simulink model "DC_Simscape"  (R2016a)
settings: Solver=ode15s  StartTime=0.0  StopTime=10  RelTol=1e-3
PreLoadFcn:
  | t_sim = 1;
  | T = 25;
libraries: fl_lib x6, nesl_utility x5, simulink x4, elec_lib x1
Description:
  | Schottky Barrier Diode Characteristics
  | 
  | This example shows generation of the current versus voltage curve
  | for a Schottky barrier diode. Define the vector of temperatures for
  | which to plot the characteristics by double clicking on the block
  | labeled 'Define temperatures'. Then double click on the block
  | labeled 'Generate Characteristics'. The datasheet for this device
  | gives Vf = 0.4V when If = 10mA, and Vf = 0.65V when If = 100mA.
  | The ohmic resistance is set to one over the gradient of the
  | datasheet I-V curve at higher voltages. The temperature
  | dependence is then modeled by selecting the default energy gap
  | and saturation current temperature exponent values for a Schottky
  | barrier diode. The plot produced by this test model can be used to
  | validate the implementation against the datasheet I-V plots.
  | 
  | 
  | Copyright 2008-2016 The MathWorks, Inc.
settings Model: ExtModeAutoUpdateStatusClock=off  Creator=MathWorks  LastModifiedBy=sara
settings DataIOCC: LimitDataPoints=on  SaveFormat=Array  SignalLoggingSaveFormat=ModelDataLogs  OutputOption=SpecifiedOutputTimes  OutputTimes=[0:t_sim/4000:t_sim]  Refine=5
settings OptimizationCC: ExpressionDepthLimit=2147483647  InitFltsAndDblsToZero=on
settings DebuggingCC: SaveWithParameterizedLinksMsg=none  UnderspecifiedInitializationDetection=Classic  MergeDetectMultiDrivingBlocksExec=none  SignalResolutionControl=TryResolveAllWithWarning  FcnCallInpInsideContextMsg=UseLocalSettings  StateNameClashWarn=warning
settings HardwareCC: ProdBitPerPointer=32  ProdLargestAtomicFloat=None  ProdIntDivRoundTo=Undefined  ProdEndianess=Unspecified  ProdWordSize=32  ProdHWDeviceType=32-bit Generic
settings ModelReferenceCC: PropagateSignalLabelsOutOfModel=off
settings GRTTargetCC: TargetFcnLib=ansi_tfl_tmw.mat  CombineOutputUpdateFcns=off  GRTInterface=on
settings ConfigComp: CovModelRefEnable=Off  CovSFcnEnable=off

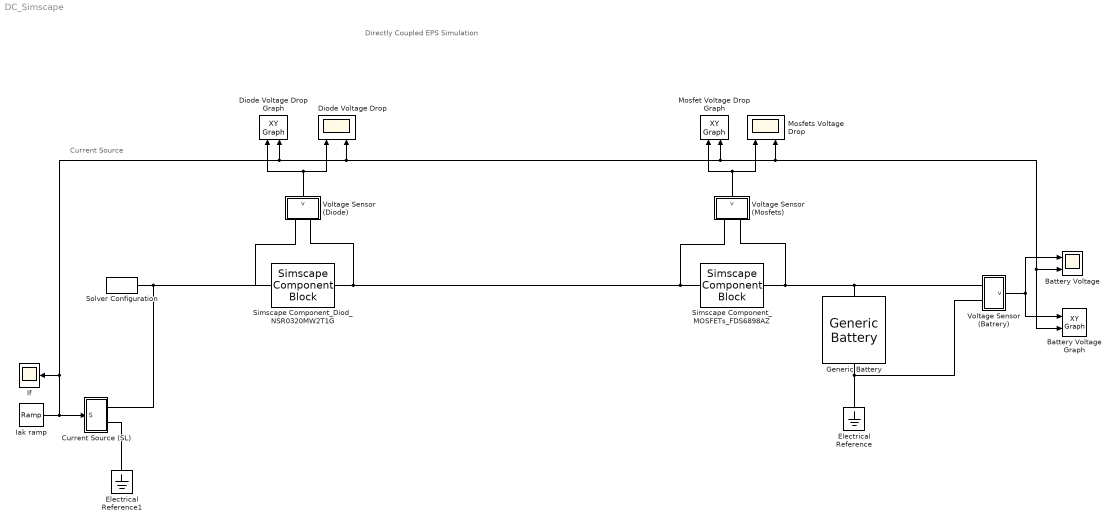
== system DC_Simscape ==
  note: Current Source
  note: Directly Coupled EPS Simulation
  " Mosfet Voltage Drop Graph" : simulink/Sinks/XY Graph  xmin=0  xmax=1  ymin=0  ymax=1  st=-1
  Battery Voltage : Scope  NumInputPorts=2
  Battery Voltage Graph : simulink/Sinks/XY Graph  xmin=0  xmax=10  ymin=0  ymax=3  st=-1
  Current Source (SL) : Subsystem
      settings: CopyFcn=set_param(gcb,'LinkStatus','none')
  Diode Voltage Drop : Scope  NumInputPorts=2
  Diode Voltage Drop Graph : simulink/Sinks/XY Graph  xmin=0  xmax=1  ymin=0  ymax=1  st=-1
  Electrical Reference : fl_lib/Electrical/Electrical Elements/Electrical Reference
  Electrical Reference1 : fl_lib/Electrical/Electrical Elements/Electrical Reference
  Generic Battery : elec_lib/Sources/Generic Battery  Vnom=2 V  R1=2 Ohm  prm_AH=1  AH=50 hr*A  AH0=50 hr*A  V1=11.5 V  AH1=25 hr*A  prm_R2=1  R2=2e+3 Ohm
  Iak ramp : simulink/Sources/Ramp  slope=2  start=0  X0=0.01
  If : Scope
  Mosfets Voltage Drop : Scope  NumInputPorts=2
  Simscape Component_Diod_NSR0320MW2T1G : SimscapeComponentBlock  SourceFile=diode_EPS  ComponentPath=diode_EPS  ComponentVariants=diode_EPS  ComponentVariantNames=diode_EPS  ClassName=diode_EPS  SchemaVersion=1  Vt=1.38e-23 * 298 / 1.60e-19 V  R=0.0084 Ohm  n=1.00404  Is=1.3032e-6 A  i_specify=off  i_priority=None  i=1 A  v_specify=off  v_priority=None  v=0 V
      settings: CopyFcn=simscape.engine.sli.internal.componentblockcallback(gcbh,'COPY')  PreCopyFcn=simscape.engine.sli.internal.componentblockcallback(gcbh,'PRECOPY')  PreDeleteFcn=simscape.engine.sli.internal.componentblockcallback(gcbh,'PREDELETE')
      mask Type: Code produced by Embedded Systems Group - UFSC
      mask Display:
      | disp('Simscape\n\n\n')
      | disp('\n\n\ndiode_EPS');
      | color('red');
      | port_label('RConn', 1,'-');
      | port_label('LConn', 1,'+');
  Simscape Component_MOSFETs_FDS6898AZ : SimscapeComponentBlock  SourceFile=MOSFETs_EPS  ComponentPath=MOSFETs_EPS  ComponentVariants=MOSFETs_EPS  ComponentVariantNames=MOSFETs_EPS  ClassName=MOSFETs_EPS  SchemaVersion=1  Vt=1.38e-23 * 298 / 1.60e-19 V  Rsd=0.27 Ohm  Rs=0.008235 Ohm  n=1.89492  Is=1.26064e-7 A  i_specify=off  i_priority=None  i=1 A  v_specify=off  v_priority=None  v=0 V  Vr_DC_specify=off  Vr_DC_priority=None  Vr_DC=0 V  Vr_CC_specify=off  Vr_CC_priority=None  Vr_CC=0 V
      settings: CopyFcn=simscape.engine.sli.internal.componentblockcallback(gcbh,'COPY')  PreCopyFcn=simscape.engine.sli.internal.componentblockcallback(gcbh,'PRECOPY')  PreDeleteFcn=simscape.engine.sli.internal.componentblockcallback(gcbh,'PREDELETE')
      mask Type: Code produced by Embedded Systems Group - UFSC
      mask Display:
      | disp('Simscape\n\n\n')
      | disp('\n\n\nMOSFETs_EPS');
      | color('red');
      | port_label('RConn', 1,'-');
      | port_label('LConn', 1,'+');
  Solver Configuration : nesl_utility/Solver Configuration  PhysicalDomain=network_engine_domain  SubClassName=solver  LeftPortType=input  RightPortType=generic  Accelerate=off  Tones=[]  Harmonics=[]  SimulateNoise=off  Profile=off  UseLocalSampling=off  EnableSwitchedLinearOptims=on  FrequencyDomain=off  UseCCode=off  RelTol=0.001  AbsTol=1e-06  MinStep=1e-09  ToWorkspace=off  RevertToSquareIcSolve=off  NumHomotopyIterations=100  PhasorMode=off  PhasorModeNumHarmonics=1  OverrideAbsTol=off  DoDC=on  ResidualTolerance=1e-9  UseLocalSolver=off  LocalSolverChoice=NE_BACKWARD_EULER_ADVANCER  LocalSolverSampleTime=.001  DoFixedCost=off  MaxNonlinIter=3  MaxModeIter=2  LinearAlgebra=Sparse  DelaysMemoryBudget=1024  AutomaticFiltering=on  FilteringTimeConstant=0.001
  Voltage Sensor (Batrery) : Subsystem
      settings: CopyFcn=set_param(gcb,'LinkStatus','none')
  Voltage Sensor (Diode) : Subsystem
      settings: CopyFcn=set_param(gcb,'LinkStatus','none')
  Voltage Sensor (Mosfets) : Subsystem
      settings: CopyFcn=set_param(gcb,'LinkStatus','none')
  wires:
  Voltage Sensor (Mosfets)/1(v) -> " Mosfet Voltage Drop Graph"/1, Mosfets Voltage Drop/1
  Voltage Sensor (Batrery)/1(v) -> Battery Voltage Graph/1, Battery Voltage/1
  Iak ramp/1 -> Current Source (SL)/1(S), Battery Voltage/2, Battery Voltage Graph/2, Mosfets Voltage Drop/2, " Mosfet Voltage Drop Graph"/2, Diode Voltage Drop/2, Diode Voltage Drop Graph/2, If/1
  Voltage Sensor (Diode)/1(v) -> Diode Voltage Drop Graph/1, Diode Voltage Drop/1
  connections:
  Electrical Reference1/LConn1 -- Current Source (SL)/RConn2
  Solver Configuration/RConn1 -- Simscape Component_Diod_NSR0320MW2T1G/LConn1 -- Voltage Sensor (Diode)/LConn1 -- Current Source (SL)/RConn1
  Generic Battery/LConn1 -- Voltage Sensor (Mosfets)/LConn2 -- Simscape Component_MOSFETs_FDS6898AZ/RConn1 -- Voltage Sensor (Batrery)/LConn1
  Electrical Reference/LConn1 -- Voltage Sensor (Batrery)/LConn2 -- Generic Battery/RConn1
  Voltage Sensor (Diode)/LConn2 -- Simscape Component_MOSFETs_FDS6898AZ/LConn1 -- Voltage Sensor (Mosfets)/LConn1 -- Simscape Component_Diod_NSR0320MW2T1G/RConn1

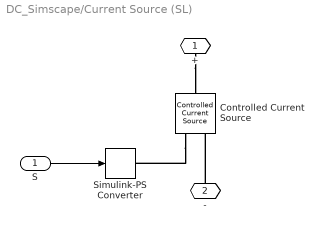
== system DC_Simscape/Current Source (SL) ==
  S : Inport
  Controlled Current Source : fl_lib/Electrical/Electrical Sources/Controlled Current Source
  Simulink-PS Converter : nesl_utility/Simulink-PS Converter  PhysicalDomain=network_engine_domain  SubClassName=ps_input  LeftPortType=input  RightPortType=output  PseudoPeriodic=off  Frequencies=[]  NoiseDistribution=none  NoiseParameters=[]  Unit=A  AffineConversion=off  InputFiltering=off  SimscapeFilterOrder=1  InputFilterTimeConstant=.001  UdotUserProvided=0
  + : PMIOPort  Port=1  Side=Right
  - : PMIOPort  Port=2  Side=Right
  wires:
  S/1 -> Simulink-PS Converter/1
  connections:
  Controlled Current Source/RConn1 -- Simulink-PS Converter/RConn1
  -/RConn1 -- Controlled Current Source/RConn2
  +/RConn1 -- Controlled Current Source/LConn1

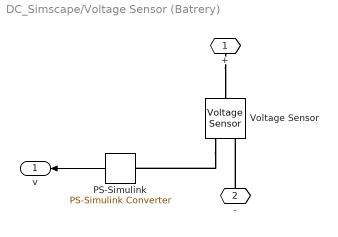
== system DC_Simscape/Voltage Sensor (Batrery) ==
  PS-Simulink : nesl_utility/PS-Simulink Converter  PhysicalDomain=network_engine_domain  SubClassName=ps_output  LeftPortType=input  RightPortType=output  PseudoPeriodic=off  Frequencies=[]  Unit=V  AffineConversion=off
  Voltage Sensor : fl_lib/Electrical/Electrical Sensors/Voltage Sensor
  + : PMIOPort  Port=1  Side=Left
  - : PMIOPort  Port=2  Side=Left
  v : Outport
  wires:
  PS-Simulink/1 -> v/1
  connections:
  -/RConn1 -- Voltage Sensor/RConn2
  +/RConn1 -- Voltage Sensor/LConn1
  Voltage Sensor/RConn1 -- PS-Simulink/LConn1

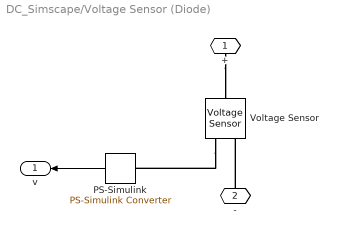
== system DC_Simscape/Voltage Sensor (Diode) ==
  PS-Simulink : nesl_utility/PS-Simulink Converter  PhysicalDomain=network_engine_domain  SubClassName=ps_output  LeftPortType=input  RightPortType=output  PseudoPeriodic=off  Frequencies=[]  Unit=V  AffineConversion=off
  Voltage Sensor : fl_lib/Electrical/Electrical Sensors/Voltage Sensor
  + : PMIOPort  Port=1  Side=Left
  - : PMIOPort  Port=2  Side=Left
  v : Outport
  wires:
  PS-Simulink/1 -> v/1
  connections:
  -/RConn1 -- Voltage Sensor/RConn2
  +/RConn1 -- Voltage Sensor/LConn1
  Voltage Sensor/RConn1 -- PS-Simulink/LConn1

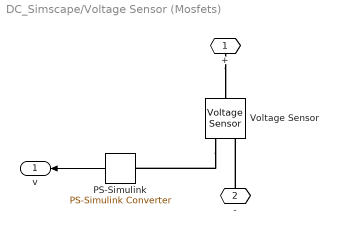
== system DC_Simscape/Voltage Sensor (Mosfets) ==
  PS-Simulink : nesl_utility/PS-Simulink Converter  PhysicalDomain=network_engine_domain  SubClassName=ps_output  LeftPortType=input  RightPortType=output  PseudoPeriodic=off  Frequencies=[]  Unit=V  AffineConversion=off
  Voltage Sensor : fl_lib/Electrical/Electrical Sensors/Voltage Sensor
  + : PMIOPort  Port=1  Side=Left
  - : PMIOPort  Port=2  Side=Left
  v : Outport
  wires:
  PS-Simulink/1 -> v/1
  connections:
  -/RConn1 -- Voltage Sensor/RConn2
  +/RConn1 -- Voltage Sensor/LConn1
  Voltage Sensor/RConn1 -- PS-Simulink/LConn1
